simulink model "relative_dist_and_velocity_plausibility_ACC"  (R2021a)
settings: Solver=VariableStepAuto  StartTime=0.0  StopTime=10.0  RelTol=1e-3
settings Model: Creator=uidk9388  LastModifiedBy=uidk9388

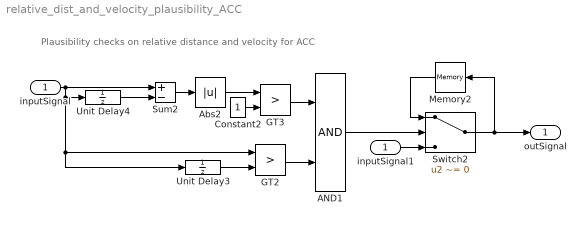
== system relative_dist_and_velocity_plausibility_ACC ==
  note: Plausibility checks on relative distance and velocity for ACC
  inputSignal : Inport
  AND1 : Logic  IconShape=distinctive  AllPortsSameDT=off  OutDataTypeStr=boolean
      mask Display: disp('AND')
  Abs2 : Abs
  Constant2 : Constant
  GT2 : RelationalOperator  Operator=>  OutDataTypeStr=boolean  RndMeth=Simplest
  GT3 : RelationalOperator  Operator=>  OutDataTypeStr=boolean  RndMeth=Simplest
  Memory2 : Memory
  Sum2 : Sum  Inputs=+-
  Switch2 : Switch  Criteria=u2 ~= 0  Threshold=0.4
  Unit Delay3 : UnitDelay  SampleTime=-1  HasFrameUpgradeWarning=on
  Unit Delay4 : UnitDelay  SampleTime=-1  HasFrameUpgradeWarning=on
  inputSignal1 : InportShadow
  outSignal : Outport
  wires:
  Unit Delay4/1 -> Sum2/2
  Constant2/1 -> GT3/2
  Memory2/1 -> Switch2/1
  inputSignal1/1 -> Switch2/3
  inputSignal/1 -> Unit Delay3/1, GT2/1, Unit Delay4/1, Sum2/1
  AND1/1 -> Switch2/2
  Switch2/1 -> Memory2/1, outSignal/1
  Sum2/1 -> Abs2/1
  Unit Delay3/1 -> GT2/2
  GT2/1 -> AND1/2
  GT3/1 -> AND1/1
  Abs2/1 -> GT3/1
